simulink model "virusPopulation"  (R2017a)
settings: Solver=VariableStepAuto  StartTime=0.0  StopTime=10.0  RelTol=1e-3
undefined symbols (not defined in the file): contractAfterSimulation, ContractAssumeBlock, contractBeforeSimulation, ContractBlock, ContractEnsureBlock, ContractGuaranteeBlock, ContractModeBlock, ContractRequireBlock, ContractValidatorBlock
libraries: Kind x6, simulink x4
settings Model: Creator=mahgoubyahia  LastModifiedBy=mahgoubyahia

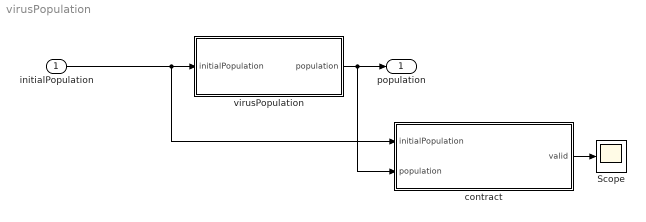
== system virusPopulation ==
  initialPopulation : Inport
  Scope : Scope
  contract : Subsystem  mask{ContractBlockType=ContractBlock}
      mask init:
      | set_param(gcb, 'LinkStatus', 'none');
      mask DialogControl DescTextVar Prompt: Contract block
      mask Display:
      | text(0.5, 0.5, '{\bf\fontsize{20}Contract}', 'hor', 'center', 'texmode','on');
      | blocks = find_system(gcb, 'LookUnderMasks','all', 'SearchDepth',1,'BlockType','Inport');
      | for i = 1 : length(blocks)
      |     blockName = get_param(blocks(i), 'Name');
      |     [path, blockName] = fileparts(char(blockName));
      |     port_label('input', i, blockName);
      | end
      | 
      | blocks = find_system(gcb, 'LookUnderMasks','all', 'SearchDepth',1,'BlockType','Outport');
      | for i = 1 : length(blocks)
      |     blockName = get_param(blocks(i), 'Name');
      |     [path, blockName] = fileparts(char(blockName));
      |     port_label('output', i, blockName);
      | end
  virusPopulation : Subsystem
  population : Outport
  wires:
  virusPopulation/1(population) -> contract/2(population), population/1
  initialPopulation/1 -> virusPopulation/1(initialPopulation), contract/1(initialPopulation)
  contract/1(valid) -> Scope/1

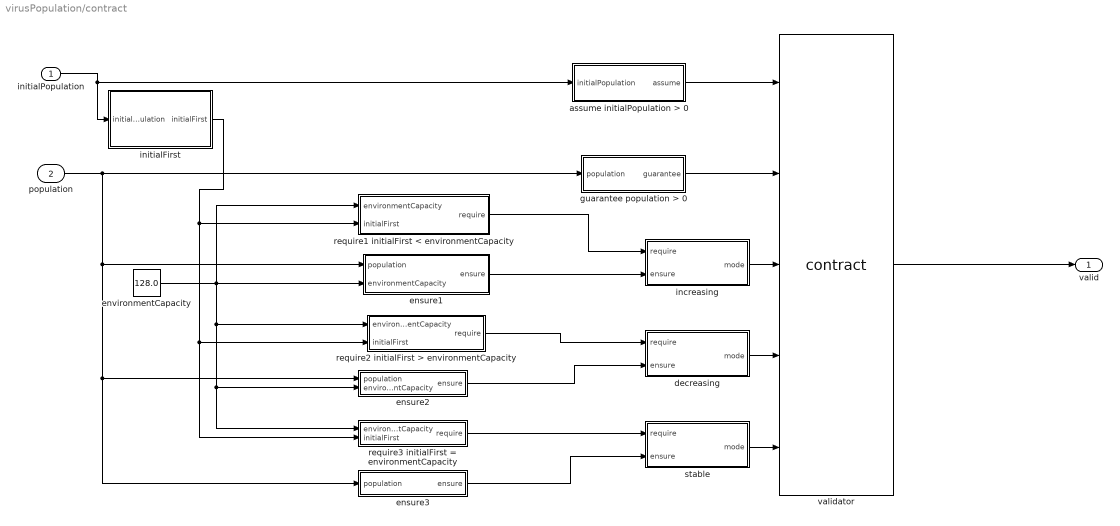
== system virusPopulation/contract ==
  initialPopulation : Inport
  population : Inport  Port=2
  assume initialPopulation > 0 : Subsystem  mask{ContractBlockType=ContractAssumeBlock}
      mask init:
      | set_param(gcb, 'LinkStatus', 'none');
      mask DialogControl DescTextVar Prompt: Assume block
  decreasing : Subsystem  mask{ContractBlockType=ContractModeBlock}
      mask init:
      | set_param(gcb, 'LinkStatus', 'none');
      mask DialogControl DescTextVar Prompt: Mode block
  ensure1 : Subsystem  mask{ContractBlockType=ContractEnsureBlock}
      mask init:
      | set_param(gcb, 'LinkStatus', 'none');
      mask DialogControl DescTextVar Prompt: Ensure block
  ensure2 : Subsystem  mask{ContractBlockType=ContractEnsureBlock}
      mask init:
      | set_param(gcb, 'LinkStatus', 'none');
      mask DialogControl DescTextVar Prompt: Ensure block
  ensure3 : Subsystem  mask{ContractBlockType=ContractEnsureBlock}
      mask init:
      | set_param(gcb, 'LinkStatus', 'none');
      mask DialogControl DescTextVar Prompt: Ensure block
  environmentCapacity : Constant  Value=128.0  OutDataTypeStr=double
  guarantee population > 0 : Subsystem  mask{ContractBlockType=ContractGuaranteeBlock}
      mask init:
      | set_param(gcb, 'LinkStatus', 'none');
      mask DialogControl DescTextVar Prompt: Guarantee block
  increasing : Subsystem  mask{ContractBlockType=ContractModeBlock}
      mask init:
      | set_param(gcb, 'LinkStatus', 'none');
      mask DialogControl DescTextVar Prompt: Mode block
  initialFirst : Subsystem
  require1 initialFirst < environmentCapacity : Subsystem  mask{ContractBlockType=ContractRequireBlock}
      mask init:
      | set_param(gcb, 'LinkStatus', 'none');
      mask DialogControl DescTextVar Prompt: Require block
  require2 initialFirst > environmentCapacity : Subsystem  mask{ContractBlockType=ContractRequireBlock}
      mask init:
      | set_param(gcb, 'LinkStatus', 'none');
      mask DialogControl DescTextVar Prompt: Require block
  require3 initialFirst = environmentCapacity : Subsystem  mask{ContractBlockType=ContractRequireBlock}
      mask init:
      | set_param(gcb, 'LinkStatus', 'none');
      mask DialogControl DescTextVar Prompt: Require block
  stable : Subsystem  mask{ContractBlockType=ContractModeBlock}
      mask init:
      | set_param(gcb, 'LinkStatus', 'none');
      mask DialogControl DescTextVar Prompt: Mode block
  validator : M-S-Function  LoadFcn=|  InitFcn=contractBeforeSimulation();  StopFcn=contractAfterSimulation();  FunctionName=contract  mask{assumePorts=1, guaranteePorts=1, modePorts=3, ContractBlockType=ContractValidatorBlock, createInportsCheckbox=on, createEnsureRequireCheckbox=on}
      | values = get_param(gcb,'MaskValues');
      | ContractValidatorBlock.block = gcb;
      | ContractValidatorBlock.assumePorts = ... 
      |     str2num(char(values(1)));
      | ContractValidatorBlock.guaranteePorts = ...
      |     str2num(char(values(2)));
      | ContractValidatorBlock.modeBlocksPorts = ...
      |     str2num(char(values(3)));
      | 
      | ContractValidatorBlock.portHandles = ...
      |     get_param(ContractValidatorBlock.block, 'PortHandles');
      | ContractValidatorBlock.portConnectivity = ...
      |     get_param(ContractValidatorBlock.block, 'PortConnectivity');
      mask prompts: assumePorts "Assume ports     :"; guaranteePorts "Guarantee ports :"; modePorts "Mode ports        :"; createInportsCheckbox "Create inports and connect them automatically"; createEnsureRequireCheckbox "Create ensure and require blocks for mode blocks"
      mask init:
      | set_param(gcb,'LinkStatus','none');
      | contract_callback('inputs_callback',gcb);
      mask DialogControl DescTextVar Prompt: The validator block implements the following logic: <br> <br> <b>Sofar</b>(assume<sub>1</sub> <b>&#8743;</b> assume<sub>2</sub> <b>&#8743;</b> ... assume<sub>k</sub>) <b>&rarr;</b> (guarantee<sub>1</sub> <b>&#8743;</b> guarantee<sub>2</sub> <b>&#8743;</b> ... guarantee<sub>m</sub> <b>&#8743;</b>  mode<sub>1</sub> <b>&#8743;</b> mode<sub>2</sub> <b>&#8743;</b> ... <b>&#8743;</b> mode<sub>n</sub> )<br> where mode<sub>i</sub> = require<sub>i</sub> <b>&rarr;</b> ensure<sub>i</sub>
      mask Display:
      | port_label('input',1,'assume')
      | port_label('input',2,'guarantee')
      | port_label('input',3,'mode')
      | port_label('input',4,'mode')
      | port_label('input',5,'mode')
      | port_label('output',1,'valid')
  valid : Outport
  wires:
  validator/1 -> valid/1
  initialPopulation/1 -> initialFirst/1(initialPopulation), assume initialPopulation > 0/1(initialPopulation)
  population/1 -> guarantee population > 0/1(population), ensure1/1(population), ensure2/1(population), ensure3/1(population)
  increasing/1(mode) -> validator/3
  require1 initialFirst < environmentCapacity/1(require) -> increasing/1(require)
  ensure1/1(ensure) -> increasing/2(ensure)
  decreasing/1(mode) -> validator/4
  require2 initialFirst > environmentCapacity/1(require) -> decreasing/1(require)
  ensure2/1(ensure) -> decreasing/2(ensure)
  stable/1(mode) -> validator/5
  require3 initialFirst = environmentCapacity/1(require) -> stable/1(require)
  ensure3/1(ensure) -> stable/2(ensure)
  guarantee population > 0/1(guarantee) -> validator/2
  assume initialPopulation > 0/1(assume) -> validator/1
  environmentCapacity/1 -> require1 initialFirst < environmentCapacity/1(environmentCapacity), ensure1/2(environmentCapacity), require3 initialFirst = environmentCapacity/1(environmentCapacity), ensure2/2(environmentCapacity), require2 initialFirst > environmentCapacity/1(environmentCapacity)
  initialFirst/1(initialFirst) -> require1 initialFirst < environmentCapacity/2(initialFirst), require2 initialFirst > environmentCapacity/2(initialFirst), require3 initialFirst = environmentCapacity/2(initialFirst)

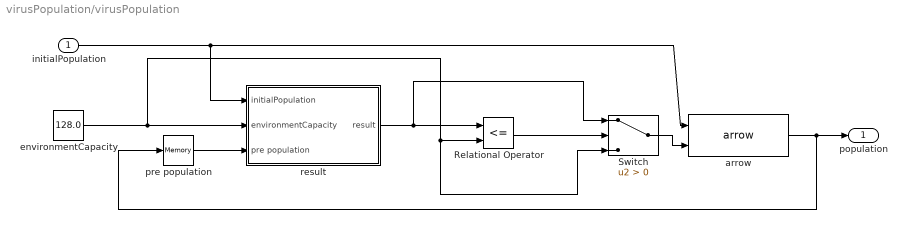
== system virusPopulation/virusPopulation ==
  initialPopulation : Inport
  Relational Operator : RelationalOperator  Operator=<=  OutDataTypeStr=boolean  RndMeth=Simplest
  Switch : Switch  Criteria=u2 > Threshold
  arrow : Kind/arrow  LustreOperatorBlock=ArrowOperator
  environmentCapacity : Constant  Value=128.0  OutDataTypeStr=double
  pre population : Memory
  result : Subsystem
  population : Outport
  wires:
  arrow/1 -> population/1, pre population/1
  Switch/1 -> arrow/2
  initialPopulation/1 -> result/1(initialPopulation), arrow/1
  environmentCapacity/1 -> result/2(environmentCapacity), Switch/3, Relational Operator/2
  pre population/1 -> result/3(pre population)
  result/1(result) -> Relational Operator/1, Switch/1
  Relational Operator/1 -> Switch/2

== system virusPopulation/contract/assume initialPopulation > 0 ==
  initialPopulation : Inport
  Compare To Zero : simulink/Logic and Bit Operations/Compare To Zero  relop=>  OutDataTypeStr=boolean
  assume : Outport  OutDataTypeStr=boolean
  wires:
  initialPopulation/1 -> Compare To Zero/1
  Compare To Zero/1 -> assume/1

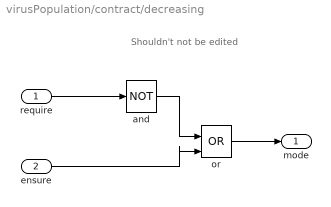
== system virusPopulation/contract/decreasing ==
  note: Shouldn't not be edited
  require : Inport  OutDataTypeStr=boolean
  ensure : Inport  Port=2  OutDataTypeStr=boolean
  and : Logic  Operator=NOT  IconShape=distinctive  AllPortsSameDT=off  OutDataTypeStr=boolean
  or : Logic  Operator=OR  IconShape=distinctive  AllPortsSameDT=off  OutDataTypeStr=boolean
  mode : Outport
  wires:
  require/1 -> and/1
  ensure/1 -> or/2
  and/1 -> or/1
  or/1 -> mode/1

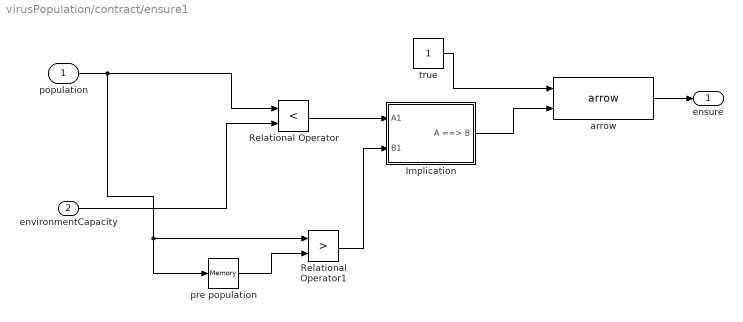
== system virusPopulation/contract/ensure1 ==
  population : Inport
  environmentCapacity : Inport  Port=2
  Implication : Subsystem  mask(CoCoSim-Implies){}
      mask help: CoCoSim block for Logical Implication
      mask Display: disp(' ')
  Relational Operator : RelationalOperator  Operator=<  OutDataTypeStr=boolean  RndMeth=Simplest
  Relational Operator1 : RelationalOperator  Operator=>  OutDataTypeStr=boolean  RndMeth=Simplest
  arrow : Kind/arrow  LustreOperatorBlock=ArrowOperator
  pre population : Memory
  true : Constant  OutDataTypeStr=boolean
  ensure : Outport  OutDataTypeStr=boolean
  wires:
  true/1 -> arrow/1
  arrow/1 -> ensure/1
  population/1 -> Relational Operator1/1, pre population/1, Relational Operator/1
  environmentCapacity/1 -> Relational Operator/2
  Relational Operator/1 -> Implication/1(A1)
  Implication/1(A ==> B) -> arrow/2
  pre population/1 -> Relational Operator1/2
  Relational Operator1/1 -> Implication/2(B1)

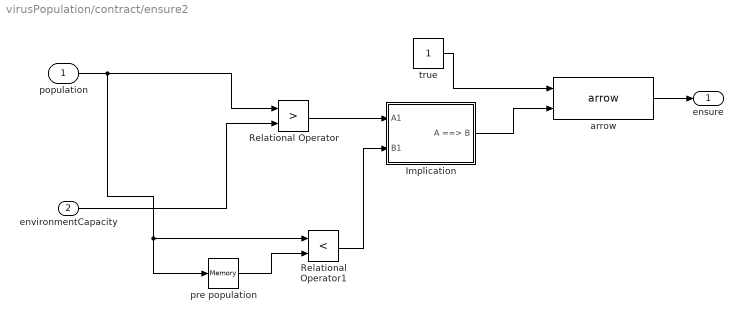
== system virusPopulation/contract/ensure2 ==
  population : Inport
  environmentCapacity : Inport  Port=2
  Implication : Subsystem  mask(CoCoSim-Implies){}
      mask help: CoCoSim block for Logical Implication
      mask Display: disp(' ')
  Relational Operator : RelationalOperator  Operator=>  OutDataTypeStr=boolean  RndMeth=Simplest
  Relational Operator1 : RelationalOperator  Operator=<  OutDataTypeStr=boolean  RndMeth=Simplest
  arrow : Kind/arrow  LustreOperatorBlock=ArrowOperator
  pre population : Memory
  true : Constant  OutDataTypeStr=boolean
  ensure : Outport  OutDataTypeStr=boolean
  wires:
  Relational Operator/1 -> Implication/1(A1)
  arrow/1 -> ensure/1
  Implication/1(A ==> B) -> arrow/2
  population/1 -> Relational Operator1/1, pre population/1, Relational Operator/1
  pre population/1 -> Relational Operator1/2
  Relational Operator1/1 -> Implication/2(B1)
  true/1 -> arrow/1
  environmentCapacity/1 -> Relational Operator/2

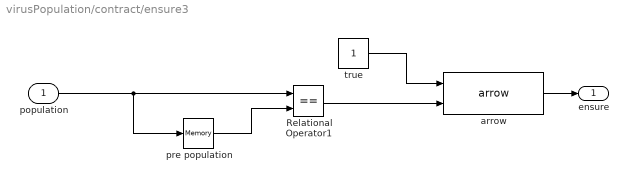
== system virusPopulation/contract/ensure3 ==
  population : Inport
  Relational Operator1 : RelationalOperator  Operator===  OutDataTypeStr=boolean  RndMeth=Simplest
  arrow : Kind/arrow  LustreOperatorBlock=ArrowOperator
  pre population : Memory
  true : Constant  OutDataTypeStr=boolean
  ensure : Outport  OutDataTypeStr=boolean
  wires:
  pre population/1 -> Relational Operator1/2
  population/1 -> pre population/1, Relational Operator1/1
  Relational Operator1/1 -> arrow/2
  true/1 -> arrow/1
  arrow/1 -> ensure/1

== system virusPopulation/contract/guarantee population > 0 ==
  population : Inport
  Compare To Zero1 : simulink/Logic and Bit Operations/Compare To Zero  relop=>  OutDataTypeStr=boolean
  guarantee : Outport  OutDataTypeStr=boolean
  wires:
  population/1 -> Compare To Zero1/1
  Compare To Zero1/1 -> guarantee/1

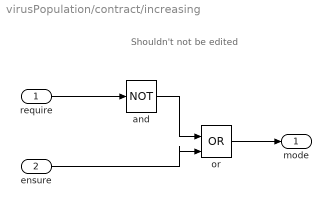
== system virusPopulation/contract/increasing ==
  note: Shouldn't not be edited
  require : Inport  OutDataTypeStr=boolean
  ensure : Inport  Port=2  OutDataTypeStr=boolean
  and : Logic  Operator=NOT  IconShape=distinctive  AllPortsSameDT=off  OutDataTypeStr=boolean
  or : Logic  Operator=OR  IconShape=distinctive  AllPortsSameDT=off  OutDataTypeStr=boolean
  mode : Outport
  wires:
  require/1 -> and/1
  ensure/1 -> or/2
  and/1 -> or/1
  or/1 -> mode/1

== system virusPopulation/contract/initialFirst ==
  initialPopulation : Inport
  arrow : Kind/arrow  LustreOperatorBlock=ArrowOperator
  pre initialFirst : Memory
  initialFirst : Outport
  wires:
  initialPopulation/1 -> arrow/1
  arrow/1 -> pre initialFirst/1, initialFirst/1
  pre initialFirst/1 -> arrow/2

== system virusPopulation/contract/require1 initialFirst < environmentCapacity ==
  environmentCapacity : Inport
  initialFirst : Inport  Port=2
  Relational Operator : RelationalOperator  Operator=<  OutDataTypeStr=boolean  RndMeth=Simplest
  require : Outport  OutDataTypeStr=boolean
  wires:
  initialFirst/1 -> Relational Operator/1
  environmentCapacity/1 -> Relational Operator/2
  Relational Operator/1 -> require/1

== system virusPopulation/contract/require2 initialFirst > environmentCapacity ==
  environmentCapacity : Inport
  initialFirst : Inport  Port=2
  Relational Operator : RelationalOperator  Operator=>  OutDataTypeStr=boolean  RndMeth=Simplest
  require : Outport  OutDataTypeStr=boolean
  wires:
  initialFirst/1 -> Relational Operator/1
  Relational Operator/1 -> require/1
  environmentCapacity/1 -> Relational Operator/2

== system virusPopulation/contract/require3 initialFirst = environmentCapacity ==
  environmentCapacity : Inport
  initialFirst : Inport  Port=2
  Relational Operator : RelationalOperator  Operator===  OutDataTypeStr=boolean  RndMeth=Simplest
  require : Outport  OutDataTypeStr=boolean
  wires:
  Relational Operator/1 -> require/1
  environmentCapacity/1 -> Relational Operator/2
  initialFirst/1 -> Relational Operator/1

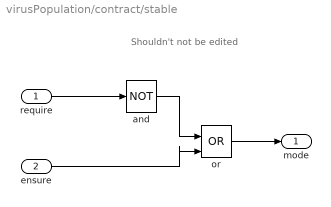
== system virusPopulation/contract/stable ==
  note: Shouldn't not be edited
  require : Inport  OutDataTypeStr=boolean
  ensure : Inport  Port=2  OutDataTypeStr=boolean
  and : Logic  Operator=NOT  IconShape=distinctive  AllPortsSameDT=off  OutDataTypeStr=boolean
  or : Logic  Operator=OR  IconShape=distinctive  AllPortsSameDT=off  OutDataTypeStr=boolean
  mode : Outport
  wires:
  require/1 -> and/1
  ensure/1 -> or/2
  and/1 -> or/1
  or/1 -> mode/1

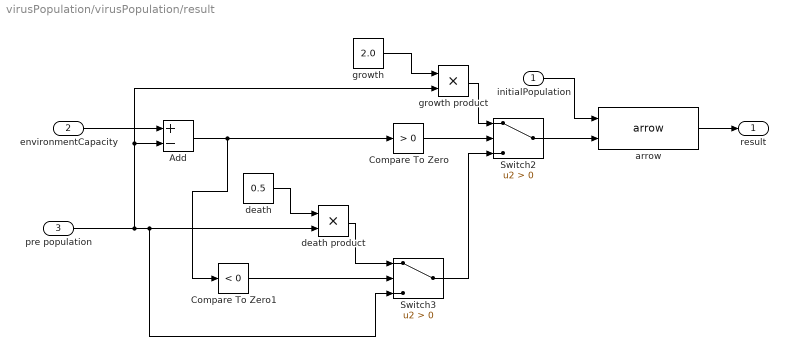
== system virusPopulation/virusPopulation/result ==
  initialPopulation : Inport
  environmentCapacity : Inport  Port=2
  pre population : Inport  Port=3
  Add : Sum  Inputs=+-
  Compare To Zero : simulink/Logic and Bit Operations/Compare To Zero  relop=>  OutDataTypeStr=boolean
  Compare To Zero1 : simulink/Logic and Bit Operations/Compare To Zero  relop=<  OutDataTypeStr=boolean
  Switch2 : Switch  Criteria=u2 > Threshold
  Switch3 : Switch  Criteria=u2 > Threshold
  arrow : Kind/arrow  LustreOperatorBlock=ArrowOperator
  death : Constant  Value=0.5  OutDataTypeStr=double
  death product : Product
  growth : Constant  Value=2.0  OutDataTypeStr=double
  growth product : Product
  result : Outport
  wires:
  Switch3/1 -> Switch2/3
  growth/1 -> growth product/1
  growth product/1 -> Switch2/1
  Compare To Zero1/1 -> Switch3/2
  pre population/1 -> Switch3/3, death product/2, Add/2, growth product/2
  Compare To Zero/1 -> Switch2/2
  death/1 -> death product/1
  environmentCapacity/1 -> Add/1
  death product/1 -> Switch3/1
  Add/1 -> Compare To Zero1/1, Compare To Zero/1
  Switch2/1 -> arrow/2
  arrow/1 -> result/1
  initialPopulation/1 -> arrow/1

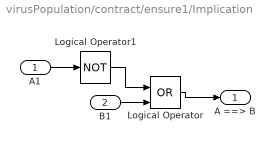
== system virusPopulation/contract/ensure1/Implication ==
  A1 : Inport
  B1 : Inport  Port=2
  Logical Operator : Logic  Operator=OR  IconShape=distinctive  AllPortsSameDT=off  OutDataTypeStr=boolean
  Logical Operator1 : Logic  Operator=NOT  IconShape=distinctive  AllPortsSameDT=off  OutDataTypeStr=boolean
  A ==> B : Outport
  wires:
  A1/1 -> Logical Operator1/1
  Logical Operator1/1 -> Logical Operator/1
  B1/1 -> Logical Operator/2
  Logical Operator/1 -> A ==> B/1

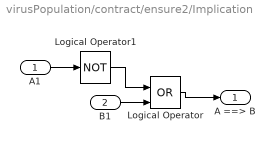
== system virusPopulation/contract/ensure2/Implication ==
  A1 : Inport
  B1 : Inport  Port=2
  Logical Operator : Logic  Operator=OR  IconShape=distinctive  AllPortsSameDT=off  OutDataTypeStr=boolean
  Logical Operator1 : Logic  Operator=NOT  IconShape=distinctive  AllPortsSameDT=off  OutDataTypeStr=boolean
  A ==> B : Outport
  wires:
  A1/1 -> Logical Operator1/1
  Logical Operator1/1 -> Logical Operator/1
  B1/1 -> Logical Operator/2
  Logical Operator/1 -> A ==> B/1
